simulink model "pendulumOnACart"  (R2013b)
settings: Solver=ode45  StartTime=0.0  StopTime=20  RelTol=1e-3
InitFcn:
  | pendulumOnACart_init;
values from neighbouring files (symbols this model uses):
  C = [1  0  0  0 ... (first row only)    [pendulumOnACart_MIMO_init.m]    (also in pendulumOnACart_disturbance_rejection_init.m; pendulumOnACart_observer_MIMO_init.m; pendulumOnACart_observer_PD_init.m)
  cM = 5    [pendulumOnACart_MIMO_init.m]    (also in pendulumOnACart_disturbance_rejection_init.m; pendulumOnACart_observer_MIMO_init.m; pendulumOnACart_observer_PD_init.m)
  dt = 1/1000    (= 0.001)    [pendulumOnACart_MIMO_init.m]    (also in pendulumOnACart_disturbance_rejection_init.m; pendulumOnACart_observer_MIMO_init.m; pendulumOnACart_observer_PD_init.m)
  dTheta_init = 2.0    (= 2)    [pendulumOnACart_MIMO_init.m]    (also in pendulumOnACart_disturbance_rejection_init.m; pendulumOnACart_observer_MIMO_init.m; pendulumOnACart_observer_PD_init.m)
  encRez = 12    [pendulumOnACart_MIMO_init.m]    (also in pendulumOnACart_disturbance_rejection_init.m; pendulumOnACart_observer_MIMO_init.m; pendulumOnACart_observer_PD_init.m)
  fcutDeriv = 50    [pendulumOnACart_MIMO_init.m]    (also in pendulumOnACart_disturbance_rejection_init.m = 10; pendulumOnACart_observer_MIMO_init.m = 10; pendulumOnACart_observer_PD_init.m = 10)
  g = 9.81    [pendulumOnACart_MIMO_init.m]    (also in pendulumOnACart_disturbance_rejection_init.m; pendulumOnACart_observer_MIMO_init.m; pendulumOnACart_observer_PD_init.m)
  pL = 0.25    [pendulumOnACart_MIMO_init.m]    (also in pendulumOnACart_disturbance_rejection_init.m; pendulumOnACart_observer_MIMO_init.m; pendulumOnACart_observer_PD_init.m)
  pm = 1    [pendulumOnACart_MIMO_init.m]    (also in pendulumOnACart_disturbance_rejection_init.m; pendulumOnACart_observer_MIMO_init.m; pendulumOnACart_observer_PD_init.m)
  theta_init = 0.2    [pendulumOnACart_MIMO_init.m]    (also in pendulumOnACart_disturbance_rejection_init.m; pendulumOnACart_observer_MIMO_init.m; pendulumOnACart_observer_PD_init.m)
undefined symbols (not defined in the file or in its folder): kd, ki, kp
settings Model: Creator=jaustin  LastModifiedBy=jaustin

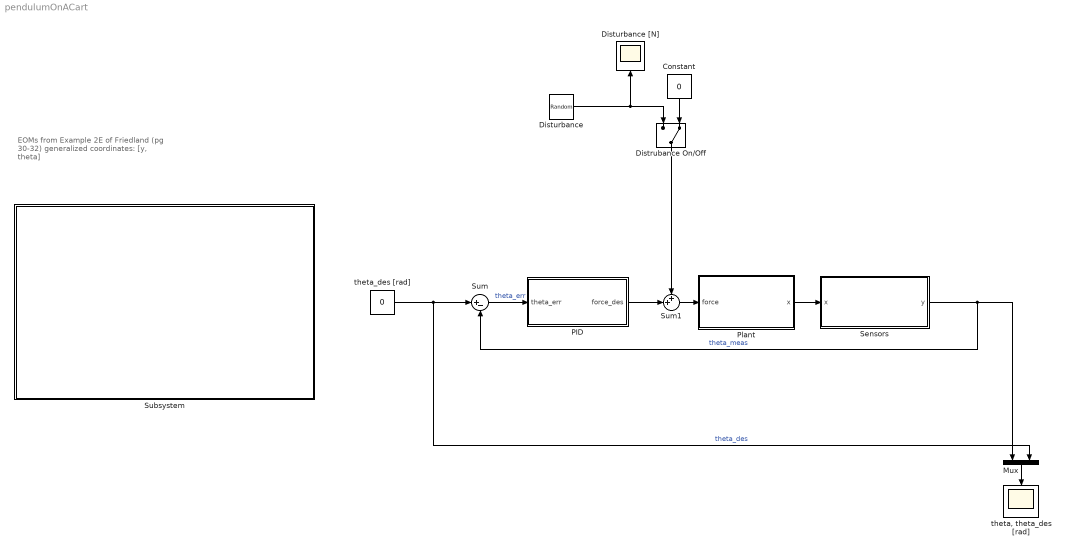
== system pendulumOnACart ==
  note: EOMs from Example 2E of Friedland
      | (pg 30-32)
      |
      | generalized coordinates: [y, theta]
  Constant : Constant  Value=0
  Distrubance On/Off : ManualSwitch  CurrentSetting=0
  Disturbance : RandomNumber  Variance=.5  SampleTime=dt*100
  Disturbance [N] : Scope
      settings: TimeRange=5  YMin=-20  YMax=80  SaveName=ScopeData7
  Mux : Mux  Inputs=2
  PID : Subsystem
  Plant : Subsystem
  Sensors : Subsystem
  Subsystem : Subsystem
      mask Display: image('pendulum_diagram.png')
  Sum : Sum  Inputs=|+-
  Sum1 : Sum  Inputs=++|
  "theta, theta_des [rad]" : Scope
      settings: TimeRange=20  YMin=-0.8  YMax=0.6000000000000001
  theta_des [rad] : Constant  Value=0
  wires:
  Mux/1 -> "theta, theta_des [rad]"/1
  Plant/1(x) -> Sensors/1(x)
  Sensors/1(y) -> Sum/2, Mux/1  "theta_meas"
  Sum1/1 -> Plant/1(force)
  Disturbance/1 -> Distrubance On/Off/1, Disturbance [N]/1
  Distrubance On/Off/1 -> Sum1/1
  Constant/1 -> Distrubance On/Off/2
  Sum/1 -> PID/1(theta_err)  "theta_err"
  theta_des [rad]/1 -> Mux/2, Sum/1  "theta_des"
  PID/1(force_des) -> Sum1/2

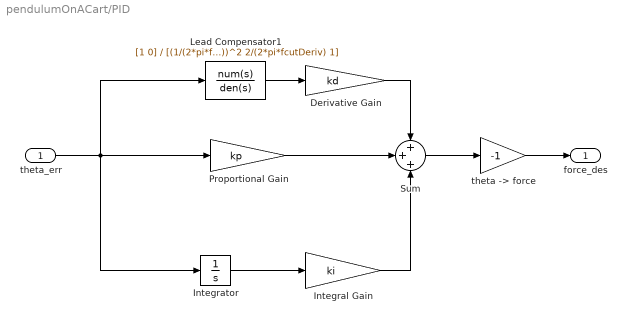
== system pendulumOnACart/PID ==
  theta_err : Inport
  Derivative Gain : Gain  Gain=kd
  Integral Gain : Gain  Gain=ki
  Integrator : Integrator  LimitOutput=on  UpperSaturationLimit=50  LowerSaturationLimit=-50
  Lead Compensator1 : TransferFcn  Numerator=[1 0]  Denominator=[(1/(2*pi*fcutDeriv))^2 2/(2*pi*fcutDeriv) 1]
  Proportional Gain : Gain  Gain=kp
  Sum : Sum  Inputs=+++
  "theta -> force" : Gain  Gain=-1
  force_des : Outport
  wires:
  Integral Gain/1 -> Sum/3
  Integrator/1 -> Integral Gain/1
  Lead Compensator1/1 -> Derivative Gain/1
  Derivative Gain/1 -> Sum/1
  Proportional Gain/1 -> Sum/2
  Sum/1 -> "theta -> force"/1
  theta_err/1 -> Lead Compensator1/1, Integrator/1, Proportional Gain/1
  "theta -> force"/1 -> force_des/1

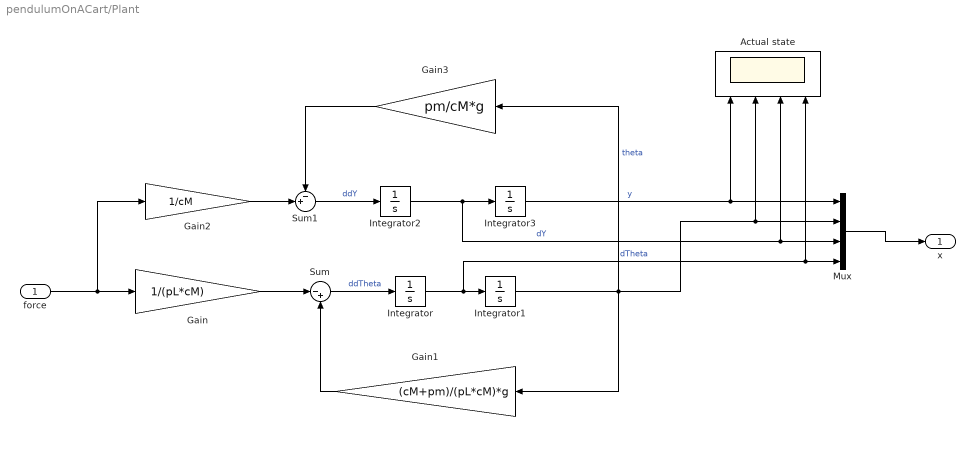
== system pendulumOnACart/Plant ==
  force : Inport
  Actual state : Scope  NumInputPorts=4
      settings: TimeRange=5  YMin=-15~-0.3~-6~-2  YMax=5~0.2~2~1  SaveName=ScopeData6
  Gain : Gain  Gain=1/(pL*cM)
  Gain1 : Gain  Gain=(cM+pm)/(pL*cM)*g
  Gain2 : Gain  Gain=1/cM
  Gain3 : Gain  Gain=pm/cM*g
  Integrator : Integrator  InitialCondition=dTheta_init
  Integrator1 : Integrator  InitialCondition=theta_init
  Integrator2 : Integrator
  Integrator3 : Integrator
  Mux : Mux
  Sum : Sum  Inputs=|-+
  Sum1 : Sum  Inputs=-+|
  x : Outport
  wires:
  Integrator1/1 -> Gain3/1, Actual state/2, Mux/2, Gain1/1  "theta"
  Gain2/1 -> Sum1/2
  Sum1/1 -> Integrator2/1  "ddY"
  Integrator2/1 -> Actual state/3, Mux/3, Integrator3/1  "dY"
  Gain/1 -> Sum/1
  force/1 -> Gain2/1, Gain/1
  Gain1/1 -> Sum/2
  Gain3/1 -> Sum1/1
  Integrator/1 -> Actual state/4, Mux/4, Integrator1/1  "dTheta"
  Sum/1 -> Integrator/1  "ddTheta"
  Mux/1 -> x/1
  Integrator3/1 -> Actual state/1, Mux/1  "y"

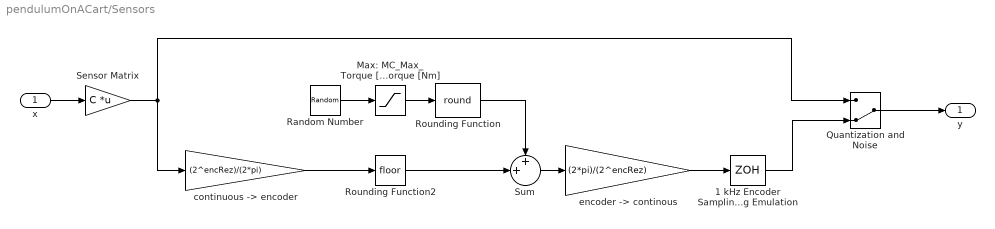
== system pendulumOnACart/Sensors ==
  x : Inport
  1 kHz Encoder Sampling Emulation : ZeroOrderHold  SampleTime=dt
  Max: MC_Max_Torque [Nm] Min: MC_Min_Torque [Nm] : Saturate  UpperLimit=1  LowerLimit=-1
  Quantization and Noise : ManualSwitch  CurrentSetting=0
  Random Number : RandomNumber  Variance=0.5  SampleTime=dt*10
  Rounding Function : Rounding  Operator=round
  Rounding Function2 : Rounding
  Sensor Matrix : Gain  Gain=C  Multiplication=Matrix(K*u)
  Sum : Sum  Inputs=++|
  "continuous -> encoder" : Gain  Gain=(2^encRez)/(2*pi)
  "encoder -> continous" : Gain  Gain=(2*pi)/(2^encRez)
  y : Outport
  wires:
  Quantization and Noise/1 -> y/1
  x/1 -> Sensor Matrix/1
  "continuous -> encoder"/1 -> Rounding Function2/1
  Rounding Function2/1 -> Sum/2
  Random Number/1 -> Max: MC_Max_Torque [Nm] Min: MC_Min_Torque [Nm]/1
  Max: MC_Max_Torque [Nm] Min: MC_Min_Torque [Nm]/1 -> Rounding Function/1
  Sum/1 -> "encoder -> continous"/1
  Rounding Function/1 -> Sum/1
  "encoder -> continous"/1 -> 1 kHz Encoder Sampling Emulation/1
  1 kHz Encoder Sampling Emulation/1 -> Quantization and Noise/2
  Sensor Matrix/1 -> Quantization and Noise/1, "continuous -> encoder"/1

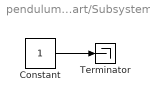
== system pendulumOnACart/Subsystem ==
  Constant : Constant
  Terminator : Terminator
  wires:
  Constant/1 -> Terminator/1
